simulink model "PIDScreenCapture"  (R2020b)
settings: Solver=VariableStepAuto  StartTime=0.0  StopTime=10.0  RelTol=1e-3
undefined symbols (not defined in the file or in its folder): daq, Kd, Ki, Kp, Kw, pid
settings Model: Creator=Utente  LastModifiedBy=Utente

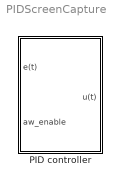
== system PIDScreenCapture ==
  "PID controller " : Subsystem

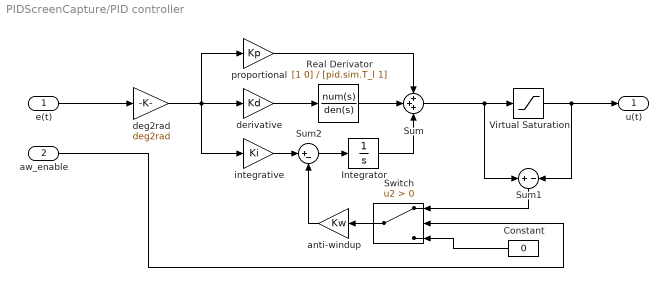
== system PIDScreenCapture/PID controller  ==
  e(t) : Inport  Unit=deg
  aw_enable : Inport  Port=2  Unit=deg
  Constant : Constant  Value=0
  Integrator : Integrator
  Real Derivator : TransferFcn  Numerator=[1 0]  Denominator=[pid.sim.T_l 1]
  Sum : Sum  Inputs=+++
  Sum1 : Sum  Inputs=+|-
  Sum2 : Sum  Inputs=|+-
  Switch : Switch  Criteria=u2 > Threshold
  Virtual Saturation : Saturate  UpperLimit=daq.dac.vdd  LowerLimit=daq.dac.vss
  anti-windup : Gain  Gain=Kw
  deg2rad : Gain  Gain=deg2rad
  derivative : Gain  Gain=Kd
  integrative : Gain  Gain=Ki
  proportional : Gain  Gain=Kp
  u(t) : Outport
  wires:
  deg2rad/1 -> integrative/1, derivative/1, proportional/1
  proportional/1 -> Sum/1
  Virtual Saturation/1 -> Sum1/2, u(t)/1
  integrative/1 -> Sum2/1
  Sum2/1 -> Integrator/1
  anti-windup/1 -> Sum2/2
  Integrator/1 -> Sum/3
  Real Derivator/1 -> Sum/2
  derivative/1 -> Real Derivator/1
  aw_enable/1 -> Switch/2
  Constant/1 -> Switch/3
  Switch/1 -> anti-windup/1
  Sum1/1 -> Switch/1
  Sum/1 -> Virtual Saturation/1, Sum1/1
  e(t)/1 -> deg2rad/1
